simulink model "zad3"  (R2020b)
settings: Solver=FixedStepAuto  StartTime=0.0  StopTime=0  RelTol=1e-3
undefined symbols (not defined in the file): H, W
libraries: CPOiS_SourcesSinks x11, CPOiS_HistogramOperations x5, CPOiS_General x1, CPOiS_DataManipulation_DataTypeConversion x1
settings Model: Creator=jrybarz  LastModifiedBy=jrybarz

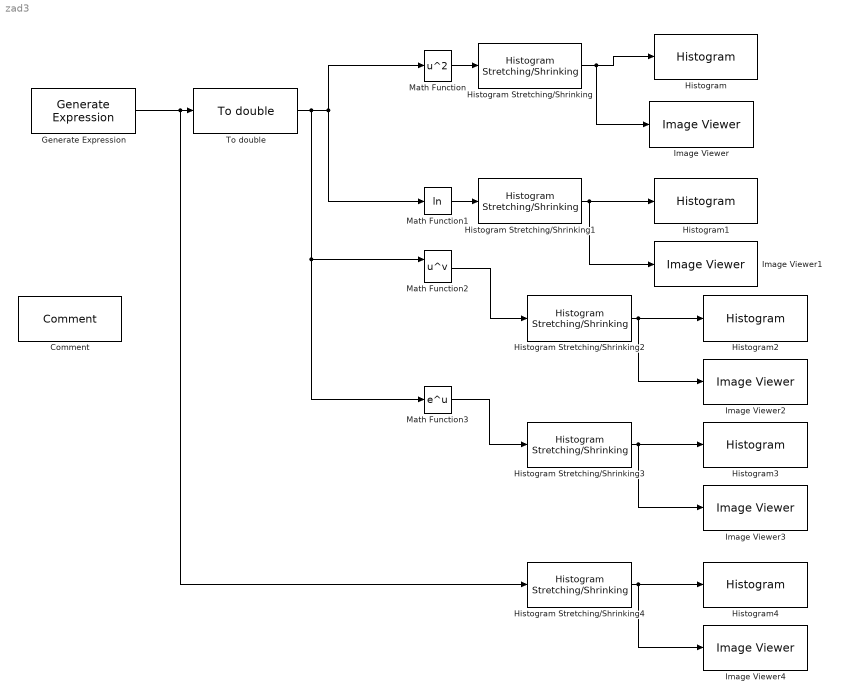
== system zad3 ==
  Comment : CPOiS_General/Comment
      settings: SourceProductName=CPOiS - Digital image and signal processing
  Generate Expression : CPOiS_SourcesSinks/Generate Expression  Width=256  Height=256  Expression=W/2+H/2
      settings: SourceProductName=CPOiS - Digital image and signal processing
  Histogram{,1..4} (5 alike) : CPOiS_SourcesSinks/Histogram
      settings: SourceProductName=CPOiS - Digital image and signal processing
  Histogram Stretching/Shrinking{,1..4} (5 alike) : CPOiS_HistogramOperations/Histogram Stretching//Shrinking  minimum=0  maximum=255
      settings: SourceProductName=CPOiS - Digital image and signal processing
  Image Viewer{,1..4} (5 alike) : CPOiS_SourcesSinks/Image Viewer
      settings: SourceProductName=CPOiS - Digital image and signal processing
  Math Function : Math  Operator=square  SaturateOnIntegerOverflow=on
  Math Function1 : Math  Operator=log  SaturateOnIntegerOverflow=on
  Math Function2 : Math  Operator=pow  SaturateOnIntegerOverflow=on
  Math Function3 : Math  SaturateOnIntegerOverflow=on
  To double : CPOiS_DataManipulation_DataTypeConversion/To double
      settings: SourceProductName=CPOiS - Digital image and signal processing
  wires:
  Math Function1/1 -> Histogram Stretching/Shrinking1/1
  Math Function/1 -> Histogram Stretching/Shrinking/1
  Histogram Stretching/Shrinking/1 -> Image Viewer/1, Histogram/1
  Histogram Stretching/Shrinking1/1 -> Image Viewer1/1, Histogram1/1
  Generate Expression/1 -> Histogram Stretching/Shrinking4/1, To double/1
  To double/1 -> Math Function3/1, Math Function2/1, Math Function/1, Math Function1/1
  Histogram Stretching/Shrinking2/1 -> Image Viewer2/1, Histogram2/1
  Histogram Stretching/Shrinking3/1 -> Image Viewer3/1, Histogram3/1
  Histogram Stretching/Shrinking4/1 -> Image Viewer4/1, Histogram4/1
  Math Function2/1 -> Histogram Stretching/Shrinking2/1
  Math Function3/1 -> Histogram Stretching/Shrinking3/1
